simulink model "rtmc_cms"  (R2014b)
settings: Solver=ode45  StartTime=0.0  StopTime=30  RelTol=1e-3
undefined symbols (not defined in the file): active_axes
libraries: vrlib x3, simulink x1
settings Model: Creator=mkatliar  LastModifiedBy=mkatliar

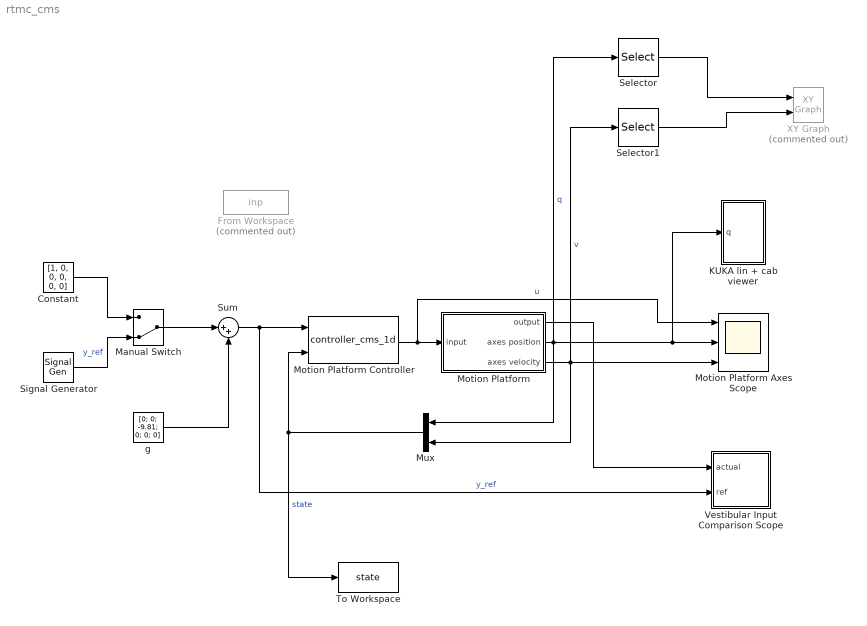
== system rtmc_cms ==
  Constant : Constant  Value=[1, 0, 0, 0, 0, 0]
  From Workspace : FromWorkspace  Commented=on  VariableName=inp  SampleTime=0
  KUKA lin + cab viewer : Subsystem
  Manual Switch : ManualSwitch  CurrentSetting=0
  Motion Platform : Subsystem  mask{q0=[4.0 1.5708   -1.5319    0.4760    0    0.1396  0    0.7991], v0=[0, 0, 0, 0, 0, 0, 0, 0], nq=[0.0, 0.0, 0.0, 0.0, 0.0, 0.0, 0.0, 0.0], nv=[0.0, 0.0, 0.0, 0.0, 0.0, 0.0, 0.0, 0.0]}
      mask prompts: q0 "Initial Axes Position"; v0 "Initial Axes Velocity"; nq "Position Sensor Noise"; nv "Velocity Sensor Noise"
  Motion Platform Axes Scope : Scope  NumInputPorts=3
      settings: TimeRange=23.988  YMin=-1~-2~-0.35  YMax=1.5~5~0.05  ScrollMode=on
  Motion Platform Controller : S-Function  FunctionName=controller_cms_1d  Parameters=qMin qMax vMin vMax uMin uMax washoutPos washoutFactor nIntervals errorWeight finalVelocityZero  EnableBusSupport=off  mask{qMin=[0.2000       -Inf    -2.1447    -0.7540    -3.0159    -0.8727    -3.0159     0.5700], qMax=[9.3000        Inf    -0.8727     1.5415     3.0159     0.8727     3.0159     1.1603], vMin=[-1.4700, -1.1802, -0.9749, -1.1802, -1.2999, -1.2999, -2.0525, -0.2450] .* active_axes, vMax=[1.4700, 1.1802, 0.9749, 1.1802, 1.2999, 1.2999, 2.0525, 0.2450] .* active_axes, uMin=[-1.0780    -1.6762    -1.1973    -2.1893    -0.5644    -1.6249    -1.3170    -0.9800], uMax=[1.0780     1.6762     1.1973     2.1893     0.5644     1.6249     1.3170     0.9800], washoutPos=[4.0 1.5708   -1.5319    0.4760    0    0.1396  0    0.7991], washoutFactor=0, nIntervals=100, finalVelocityZero=off, errorWeight=[1, 1, 1, 1, 1, 1]}
      mask prompts: qMin "Position Min"; qMax "Position Max"; vMin "Velocity Min"; vMax "Velocity Max"; uMin "Acceleration Min"; uMax "Acceleration Max"; washoutPos "Position"; washoutFactor "Factor"; nIntervals "Number of Intervals"; finalVelocityZero "Final Velocity Zero"; errorWeight "Error Weight"
  Mux : Mux  Inputs=2
  Selector : Selector  InputPortWidth=8
  Selector1 : Selector  InputPortWidth=8
  Signal Generator : SignalGenerator  Amplitude=[1, 0, 0, 0, 0, 0]
  Sum : Sum  Inputs=|++
  To Workspace : ToWorkspace  VariableName=state  SaveFormat=Timeseries  SampleTime=-1
  Vestibular Input Comparison Scope : Subsystem
  XY Graph : simulink/Sinks/XY Graph  Commented=on  xmin=-1  xmax=1  ymin=-1  ymax=1  st=-1
  g : Constant  Value=[0; 0; -9.81; 0; 0; 0]
  wires:
  Motion Platform Controller/1 -> Motion Platform Axes Scope/1, Motion Platform/1(input)  "u"
  Sum/1 -> Motion Platform Controller/1, Vestibular Input Comparison Scope/2(ref)  "y_ref"
  g/1 -> Sum/2
  Signal Generator/1 -> Manual Switch/2  "y_ref"
  Motion Platform/2(axes position) -> Selector/1, Mux/1, KUKA lin + cab viewer/1(q), Motion Platform Axes Scope/2  "q"
  Motion Platform/1(output) -> Vestibular Input Comparison Scope/1(actual)
  Mux/1 -> Motion Platform Controller/2, To Workspace/1  "state"
  Motion Platform/3(axes velocity) -> Selector1/1, Mux/2, Motion Platform Axes Scope/3  "v"
  Selector/1 -> XY Graph/1
  Selector1/1 -> XY Graph/2
  Constant/1 -> Manual Switch/1
  Manual Switch/1 -> Sum/1

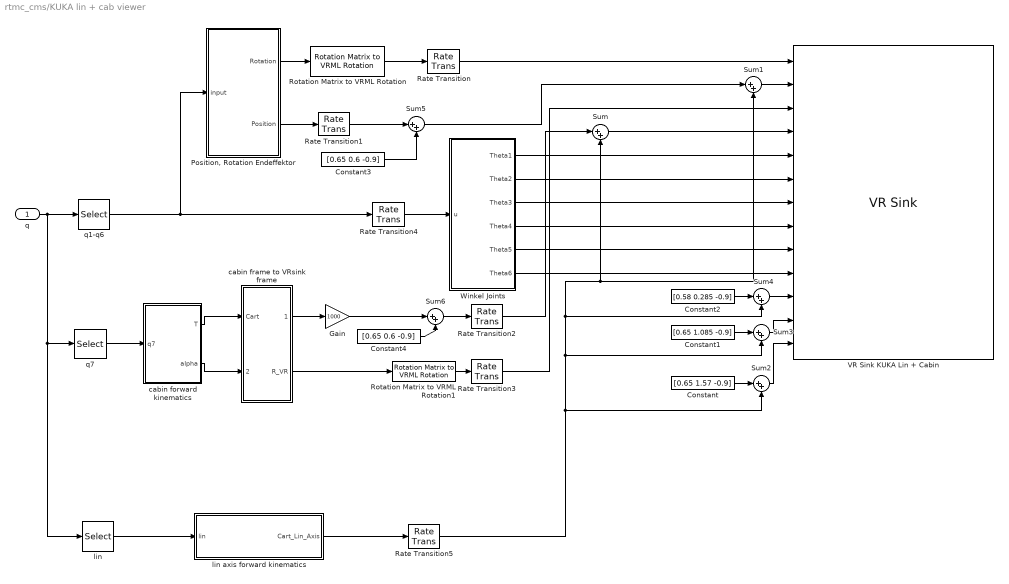
== system rtmc_cms/KUKA lin + cab viewer ==
  q : Inport
  Constant : Constant  Value=[0.65 1.57 -0.9]
  Constant1 : Constant  Value=[0.65 1.085 -0.9]
  Constant2 : Constant  Value=[0.58 0.285 -0.9]
  Constant3 : Constant  Value=[0.65 0.6 -0.9]
  Constant4 : Constant  Value=[0.65 0.6 -0.9]
  Gain : Gain  Gain=1000
  "Position, Rotation Endeffektor" : MATLAB Function  TreatAsAtomicUnit=on
  Rate Transition{,1..5} (6 alike) : RateTransition
  Rotation Matrix to VRML Rotation : vrlib/Utilities/Rotation Matrix to VRML Rotation  maxzero=1e-12
  Rotation Matrix to VRML Rotation1 : vrlib/Utilities/Rotation Matrix to VRML Rotation  maxzero=1e-12
  Sum{,1..6} (7 alike) : Sum  Inputs=|++
  VR Sink KUKA Lin + Cabin : vrlib/VR Sink  InstantiateOnLoad=on  SampleTime=0.1  ViewEnable=on  RemoteChange=off  RemoteView=on  FieldsWritten=Mount.rotation.4.1.double#Mount.translation.3.1.double#Cabin.rotation.4.1.double#Cabin.translation.3.1.double#AXIS_04_OBJ.rotation.4.1.double#AXIS_27_OBJ.rotation.4.1.double#AXIS_32_OBJ.rotation.4.1.double#AXIS_44_OBJ.rotation.4.1.double#AXIS_46_OBJ.rotation.4.1.double#AXIS_49_OBJ.rotation.4.1.double#Sled.translation.3.1.double#Tonne.translation.3.1.double#KR500.translation.3.1.double  WorldFileName=kr500_cabin_linear.wrl  AutoView=off  VideoDimensions=[]  AllowVariableSize=off  FigureProperties="{'Position', 'Name', 'Viewpoint', 'CameraBound', 'CameraDirection', 'CameraPosition', 'CameraUpVector', 'ZoomFactor', 'Antialiasing', 'Headlight', 'Lighting', 'NavPanel', 'Sound', 'StatusBar', 'Stereo3D', 'Stereo3DCameraOffset', 'Stereo3DHIT', 'ToolBar', 'Textures', 'Transparency', 'Triad', 'Wireframe', 'NavZones', 'NavMode', 'NavSpeed', 'CaptureFileFormat', 'CaptureFileName', 'Record2DCompressMethod', 'Record2DCompressQuality', 'Record2D', 'Record2DFileName', 'Record2DFPS'; [1.3230000000000000e+03   6.9100000000000000e+02   5.7600000000000000e+02   3.8000000000000000e+02], '', 'from Top', 'on', [0.0000000000000000e+00   0.0000000000000000e+00  -1.0000000000000000e+00], [0.0000000000000000e+00   0.0000000000000000e+00   0.0000000000000000e+00], [0.0000000000000000e+00   1.0000000000000000e+00   0.0000000000000000e+00], [1.0000000000000000e+00], 'on', 'on', 'on', 'halfbar', 'on', 'on', 'off', [1.0000000149011612e-01], [0.0000000000000000e+00], 'on', 'on', 'on', 'none', 'off', 'off', 'fly', 'normal', 'tif', '%f_anim_%n.tif', 'auto', [7.5000000000000000e+01], 'off', '%f_anim_%n.avi', 'auto'}"
  Winkel Joints : MATLAB Function  TreatAsAtomicUnit=on
  cabin forward kinematics : MATLAB Function  TreatAsAtomicUnit=on
  cabin frame to VRsink frame : MATLAB Function  TreatAsAtomicUnit=on
  lin : Selector  InputPortWidth=8
  lin axis forward kinematics : MATLAB Function  TreatAsAtomicUnit=on
  q1-q6 : Selector  InputPortWidth=8  Indices=2:7
  q7 : Selector  InputPortWidth=8  Indices=8
  wires:
  Constant4/1 -> Sum6/2
  Gain/1 -> Sum6/1
  Sum6/1 -> Rate Transition2/1
  Constant3/1 -> Sum5/2
  Rate Transition1/1 -> Sum5/1
  Sum5/1 -> Sum1/1
  Constant2/1 -> Sum4/1
  Sum4/1 -> VR Sink KUKA Lin + Cabin/11
  Constant1/1 -> Sum3/1
  Sum3/1 -> VR Sink KUKA Lin + Cabin/12
  Constant/1 -> Sum2/1
  Sum2/1 -> VR Sink KUKA Lin + Cabin/13
  Sum1/1 -> VR Sink KUKA Lin + Cabin/2
  Sum/1 -> VR Sink KUKA Lin + Cabin/4
  lin axis forward kinematics/1(Cart_Lin_Axis) -> Rate Transition5/1
  Rate Transition5/1 -> Sum4/2, Sum1/2, Sum/2, Sum3/2, Sum2/2
  cabin frame to VRsink frame/2(R_VR) -> Rotation Matrix to VRML Rotation1/1
  cabin frame to VRsink frame/1(Cart_VR) -> Gain/1
  cabin forward kinematics/1(T) -> cabin frame to VRsink frame/1(Cart)
  cabin forward kinematics/2(alpha) -> cabin frame to VRsink frame/2(alpha)
  Rotation Matrix to VRML Rotation1/1 -> Rate Transition3/1
  q7/1 -> cabin forward kinematics/1(q7)
  "Position, Rotation Endeffektor"/2(Position) -> Rate Transition1/1
  "Position, Rotation Endeffektor"/1(Rotation) -> Rotation Matrix to VRML Rotation/1
  Rotation Matrix to VRML Rotation/1 -> Rate Transition/1
  q1-q6/1 -> "Position, Rotation Endeffektor"/1(input), Rate Transition4/1
  q/1 -> q7/1, lin/1, q1-q6/1
  Rate Transition4/1 -> Winkel Joints/1(u)
  Rate Transition/1 -> VR Sink KUKA Lin + Cabin/1
  Winkel Joints/1(Theta1) -> VR Sink KUKA Lin + Cabin/5
  Winkel Joints/2(Theta2) -> VR Sink KUKA Lin + Cabin/6
  Winkel Joints/3(Theta3) -> VR Sink KUKA Lin + Cabin/7
  Winkel Joints/4(Theta4) -> VR Sink KUKA Lin + Cabin/8
  Winkel Joints/5(Theta5) -> VR Sink KUKA Lin + Cabin/9
  Winkel Joints/6(Theta6) -> VR Sink KUKA Lin + Cabin/10
  Rate Transition2/1 -> Sum/1
  Rate Transition3/1 -> VR Sink KUKA Lin + Cabin/3
  lin/1 -> lin axis forward kinematics/1(lin)

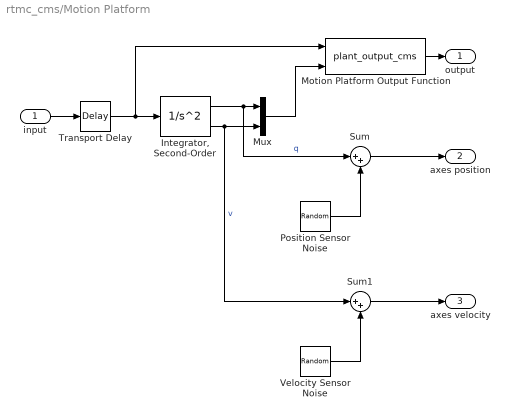
== system rtmc_cms/Motion Platform ==
  input : Inport
  "Integrator, Second-Order" : SecondOrderIntegrator  ICX=q0  ICDXDT=v0
  Motion Platform Output Function : S-Function  FunctionName=plant_output_cms  EnableBusSupport=off
  Mux : Mux  Inputs=2
  Position Sensor Noise : RandomNumber  Variance=nq.^2  SampleTime=0.012
  Sum : Sum  Inputs=|++
  Sum1 : Sum  Inputs=|++
  Transport Delay : TransportDelay  DelayTime=0.048
  Velocity Sensor Noise : RandomNumber  Variance=nv.^2  SampleTime=0.012
  output : Outport
  axes position : Outport  Port=2
  axes velocity : Outport  Port=3
  wires:
  "Integrator, Second-Order"/1 -> Sum/1, Mux/1  "q"
  "Integrator, Second-Order"/2 -> Sum1/1, Mux/2  "v"
  Motion Platform Output Function/1 -> output/1
  Transport Delay/1 -> "Integrator, Second-Order"/1, Motion Platform Output Function/1
  Mux/1 -> Motion Platform Output Function/2
  Sum/1 -> axes position/1
  Position Sensor Noise/1 -> Sum/2
  Velocity Sensor Noise/1 -> Sum1/2
  Sum1/1 -> axes velocity/1
  input/1 -> Transport Delay/1

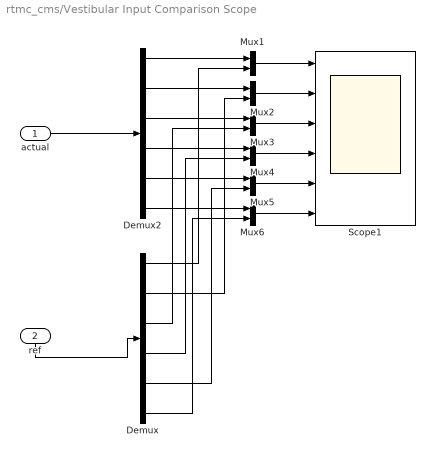
== system rtmc_cms/Vestibular Input Comparison Scope ==
  actual : Inport
  ref : Inport  Port=2
  Demux : Demux  Outputs=6
  Demux2 : Demux  Outputs=6
  Mux{1..6} (6 alike) : Mux  Inputs=2
  Scope1 : Scope  NumInputPorts=6
      settings: TimeRange=23.988  YMin=-1~-4e-06~-9.8102~-1~-1~-1  YMax=1~4e-06~-9.8098~1~1~1
  wires:
  Demux/4 -> Mux4/2
  Demux2/1 -> Mux1/1
  Demux/2 -> Mux2/2
  Demux/5 -> Mux5/2
  Mux2/1 -> Scope1/2
  Demux2/3 -> Mux3/1
  Demux2/2 -> Mux2/1
  Demux/1 -> Mux1/2
  Demux/6 -> Mux6/2
  Demux2/4 -> Mux4/1
  Demux/3 -> Mux3/2
  Demux2/6 -> Mux6/1
  Demux2/5 -> Mux5/1
  Mux1/1 -> Scope1/1
  Mux3/1 -> Scope1/3
  Mux4/1 -> Scope1/4
  Mux5/1 -> Scope1/5
  Mux6/1 -> Scope1/6
  actual/1 -> Demux2/1
  ref/1 -> Demux/1

== matlab function rtmc_cms/KUKA lin + cab viewer/Position, Rotation Endeffektor ==
  data: Rotation output; input input; Position output
function [Rotation,Position]= fcn( input )
% This block supports the Embedded MATLAB subset.
% See the help menu for details. 

Hpi = pi()/2;

Theta1 = input(1) * -1;
Theta2 = input(2);
Theta3 = input(3) - pi()/2;
Theta4 = input(4);
Theta5 = input(5);
Theta6 = input(6);
%corrections
Theta7 = Hpi;
Theta8 = -Hpi;

Trans1 = [  cos(Theta1)     -sin(Theta1)*cos(-Hpi)      sin(Theta1)*sin(-Hpi)       0.5*cos(Theta1);
            sin(Theta1)     cos(Theta1)*cos(-Hpi)       -cos(Theta1)*sin(-Hpi)      0.5*sin(Theta1);
            0               sin(-Hpi)                   cos(-Hpi)                   2.03;
            0               0                           0                           1];
Trans2 = [  cos(Theta2)     -sin(Theta2)*cos(0)         sin(Theta2)*sin(0)          1.3*cos(Theta2);
            sin(Theta2)     cos(Theta2)*cos(0)          -cos(Theta2)*sin(0)         1.3*sin(Theta2);
            0               sin(0)                      cos(0)                      0;
            0               0                           0                           1];
Trans3 = [  cos(Theta3)     -sin(Theta3)*cos(Hpi)       sin(Theta3)*sin(Hpi)        0.055*cos(Theta3);
            sin(Theta3)     cos(Theta3)*cos(Hpi)        -cos(Theta3)*sin(Hpi)       0.055*sin(Theta3);
            0               sin(Hpi)                    cos(Hpi)                    0;
            0               0                           0                           1];
Trans4 = [  cos(Theta4)     -sin(Theta4)*cos(-Hpi)      sin(Theta4)*sin(-Hpi)       0*cos(Theta4);
            sin(Theta4)     cos(Theta4)*cos(-Hpi)       -cos(Theta4)*sin(-Hpi)      0*sin(Theta4);
            0               sin(-Hpi)                   cos(-Hpi)                   -1.025;
            0               0                           0                           1];
Trans5 = [  cos(Theta5)     -sin(Theta5)*cos(Hpi)       sin(Theta5)*sin(Hpi)        0*cos(Theta5);
            sin(Theta5)     cos(Theta5)*cos(Hpi)        -cos(Theta5)*sin(Hpi)       0*sin(Theta5);
            0               sin(Hpi)                    cos(Hpi)                    0;
            0               0                           0                           1];
Trans6 = [  cos(Theta6)     -sin(Theta6)*cos(0)         sin(Theta6)*sin(0)          0*cos(Theta6);
            sin(Theta6)     cos(Theta6)*cos(0)          -cos(Theta6)*sin(0)         0*sin(Theta6);
            0               sin(0)                      cos(0)                      -0.29;
            0               0                           0                           1];
% Trans7 = [  cos(Theta7)     -sin(Theta7)*cos(Hpi)       sin(Theta7)*sin(Hpi)        0*cos(Theta7);
%             sin(Theta7)     cos(Theta7)*cos(Hpi)        -cos(Theta7)*sin(Hpi)       0*sin(Theta7);
%             0               sin(Hpi)                    cos(Hpi)                    0;
%             0               0                           0                           1];
% Trans8 = [  cos(Theta8)     -sin(Theta8)*cos(0)         sin(Theta8)*sin(0)          0*cos(Theta8);
%             sin(Theta8)     cos(Theta8)*cos(0)          -cos(Theta8)*sin(0)         0*sin(Theta8);
%             0               sin(0)                      cos(0)                      0;
%             0               0                           0                           1];

TransC = [  cos(pi)    -sin(pi)*cos(pi)       sin(pi)*sin(pi)       0*cos(pi);
            sin(pi)     cos(pi)*cos(pi)      -cos(pi)*sin(pi)       0*sin(pi);
            0           sin(pi)               cos(pi)                       0;
            0           0                     0                             1]; 
     
Rot_x = [ 1  0  0  0;
          0  0  1  0;
          0  -1 0  0;
          0  0  0  1];      
   
Fmat8 = Rot_x * Trans1 * Trans2 * Trans3 * Trans4 * Trans5 * Trans6 * TransC; %* Trans7 * Trans8    ;%verified

Position_tmp = [Fmat8(1,4) Fmat8(2,4) Fmat8(3,4) 1]';
Position = [ Position_tmp(1) Position_tmp(2) Position_tmp(3) ]';

Rot  = [ 1  0  0; ...
         0  0 -1; ...
         0  1  0];
Rot2 = [ 0  0  1; ...
         0  1  0; ...
        -1  0  0];
Rotation = Fmat8(1:3,1:3)*Rot*Rot2;

== matlab function rtmc_cms/KUKA lin + cab viewer/Winkel Joints ==
  data: u input; Theta1 output; Theta2 output; Theta3 output; Theta4 output; Theta5 output; Theta6 output
function [Theta1,Theta2,Theta3,Theta4,Theta5,Theta6]= fcn(u)
% This block supports the Embedded MATLAB subset.
% See the help menu for details. 

Theta1 = [0 1 0 u(1)];
Theta2 = [0 1 0 u(2)];
Theta3 = [0 1 0 u(3)];
Theta4 = [0 1 0 u(4)];
Theta5 = [0 1 0 u(5)];
Theta6 = [0 1 0 u(6)];

== matlab function rtmc_cms/KUKA lin + cab viewer/cabin forward kinematics ==
  data: q7 input; T output; alpha output
function [T, alpha] = fcn(q7)

d = 0.200;
Rbg = 0.504;
L = 0.570;
Rsg = 0.024;
theta = asin( (d/2)/Rbg );
q7Level = [  Rsg  (L-d)   L   (L + Rbg*(pi/2 - 2*theta))   (L + Rbg*(pi/2))   (L + Rbg*(pi/2) + L - d - Rsg)];


if (q7Level(1) <= q7) && (q7 <= q7Level(2))
    [T, alpha] = cabin_dir_kin1(q7, L, d, Rbg);
elseif (q7Level(2) <= q7) && (q7 <= q7Level(3))
    [T, alpha] = cabin_dir_kin2(q7, L, d, Rbg);
elseif (q7Level(3) <= q7) && (q7 <= q7Level(4))
    [T, alpha] = cabin_dir_kin3(q7, Rbg, q7Level, theta);
elseif (q7Level(4) <= q7) && (q7 <= q7Level(5))
    [T, alpha] = cabin_dir_kin4(q7, L, d, Rbg);
else
    [T, alpha] = cabin_dir_kin5(q7, d, Rbg, q7Level);
end
   
%=========================================================================================

% Functions for the forward kinematic of the 7th joint
function [T, alpha] = cabin_dir_kin1(q, L, d, Rbg)
    T = [ -L+q+(d/2);
           0;
           Rbg];
    alpha = 0;
    
function [T, alpha] = cabin_dir_kin2(q, L, d, Rbg)
    t271 = L^2;
    t272 = Rbg^2;
    t273 = q^2;
    t274 = d^2;
    t275 = 4*L*q*t273;
    t276 = 4*L*q*t271;
    t277 = t271^2;
    t278 = t274^2;
    t279 = 2*t271*t274;
    t280 = t273^2;
    t281 = 4*t272*t274;
    t282 = 2*t273*t274;
    t285 = 6*t271*t273;
    t286 = 4*L*q*t274;
    t283 = t275 + t276 - t277 - t278 + t279 - t280 + t281 + t282 - t285 - t286;
    t284 = t283^(1/2);
    t314 = 2*L*q;
    t287 = t271 + t272 + t273 - t314;
    t288 = abs(t287);
    t289 = 2*t271;
    t290 = 2*t272;
    t291 = 2*t273;
    t316 = 4*L*q;
    t292 = t289 + t290 + t291 - t316;
    t293 = 1/t292;
    t294 = Rbg*t284;
    t295 = L*t274;
    t296 = 3*q*t271;
    t297 = 2*q*t272;
    t310 = 2*L*t272;
    t311 = 3*L*t273;
    t312 = q*t274;
    t313 = L*t271;
    t298 = t294 + t295 + t296 + t297 - t310 - t311 - t312 - t313 + q*t273;
    t299 = t293*t298;
    t300 = L - q + t299;
    t301 = abs(t300);
    t302 = (q*t284)/2;
    t303 = t271/2;
    t304 = t274/2;
    t305 = t273/2;
    t319 = L*q;
    t306 = t303 + t304 + t305 - t319;
    t307 = Rbg*t306;
    t318 = (L*t284)/2;
    t308 = t302 + t307 - t318;
    t309 = abs(t308);
    t315 = 1/t288;
    t317 = 1/t301;
    t320 = 1/t288^2;
    t321 = 1/t301^2;
    t322 = t309^2;
    t323 = t320*t321*t322;
    t324 = t323 + 1;
    t325 = 1/t324^(1/2);
    t326 = Rbg - t293*t308;
    t327 = q/2;
    t328 = 4*t271;
    t329 = 4*t272;
    t330 = 4*t273;
    t331 = t328 + t329 + t330 - 8*L*q;
    t332 = 1/t331;
    t333 = t298*t332;
    t334 = - L/2 + t327 + t333;
    alpha = atan(t309*t315*t317);
    T = [t325*t334-t309*t315*t317*t325*t326;  0;  t325*t326+t309*t315*t317*t325*t334];
    
function [T, alpha] = cabin_dir_kin3(q, Rbg, q7Level, theta)
    alpha = theta + (q-q7Level(3))/Rbg;
    T = [ 0;
          0;
          Rbg*cos(theta)];

function [T, alpha] = cabin_dir_kin4(q, L, d, Rbg)
    t336 = 1/Rbg;
    t337 = 2*q;
    t338 = pi*Rbg;
    t343 = 2*L;
    t339 = t337 + t338 - t343;
    t340 = (t336*t339)/2;
    t341 = cos(t340);
    t342 = Rbg*t341;
    t344 = Rbg + d + t342;
    t345 = abs(t344);
    t346 = L - q;
    t347 = t336*t346;
    t355 = pi/2;
    t348 = t347 - t355;
    t349 = cos(t348);
    t350 = Rbg*t349;
    t351 = Rbg + t350;
    t352 = abs(t351);
    t353 = d - Rbg - t342;
    t354 = abs(t353);
    t356 = t345^(1/2);
    t357 = 1/t352;
    t358 = t354^(1/2);
    t359 = 1/t352^2;
    t360 = t345*t354*t359;
    t361 = t360 + 1;
    t362 = 1/t361^(1/2);
    t363 = t344^(1/2);
    t364 = t353^(1/2);
    t365 = (t363*t364)/2;
    t366 = sin(t348);
    t367 = Rbg*t366;
    t368 = t365 + t367;
    t369 = Rbg/2;
    t370 = t369 - (Rbg*t349)/2;
    alpha = atan(t356*t357*t358);
    T = [ t362*t370+t356*t357*t358*t362*t368;  0;   t356*t357*t358*t362*t370-t362*t368];
    
function [T, alpha] = cabin_dir_kin5(q, d, Rbg, q7Level)
    alpha = pi/2;
    T = [ (d/2)+q-q7Level(5);
          0; 
          Rbg];

== matlab function rtmc_cms/KUKA lin + cab viewer/cabin frame to VRsink frame ==
  data: Cart input; Cart_VR output; alpha input; R_VR output
function [Cart_VR, R_VR] = fcn(Cart, alpha)
% This block supports the Embedded MATLAB subset.
% See the help menu for details.
L = 0.570;
Rbg = 0.504;
d = 0.2;
Cart_VR = [Cart(2); Cart(3); Cart(1)] + [0; -Rbg; L-(d/2)];
R_VR = [1  0  0; 0  cos(alpha)  sin(alpha); 0  -sin(alpha)  cos(alpha)];

== matlab function rtmc_cms/KUKA lin + cab viewer/lin axis forward kinematics ==
  data: lin input; Cart_Lin_Axis output
function Cart_Lin_Axis  = fcn(lin)
% Cart_Lin_Axis = [0, 0, lin-4.9];
Cart_Lin_Axis = [0, 0, lin-9.8];
